simulink model "sistema_completo_OLD"  (R2023a)
settings: Solver=VariableStepAuto  StartTime=0.0  StopTime=2  MaxStep=1e-3  RelTol=1e-3
values from neighbouring files (symbols this model uses):
  Pp = 3    [angulo_de_desfasaje_electromagnetico.m]
  T_s_ref = 20    [Polos_ceros_Rs.m]
undefined symbols (not defined in the file or in its folder): alpha_Cu, b_eq, C_ts, J_eq, k_l, L_d, L_ls, L_q, lambda_m, omega_n_i, omega_n_pos, omega_n_v, r, R_s_ref, R_ts, tau, Vsl_max, zitta
libraries: SignalEditorBlockLib x9
settings Model: Creator=juanf  LastModifiedBy=Juan

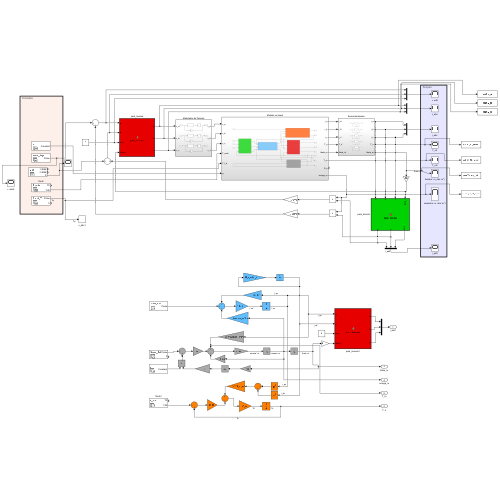
[thumbnail: Simulink's stored preview of the top-level diagram]
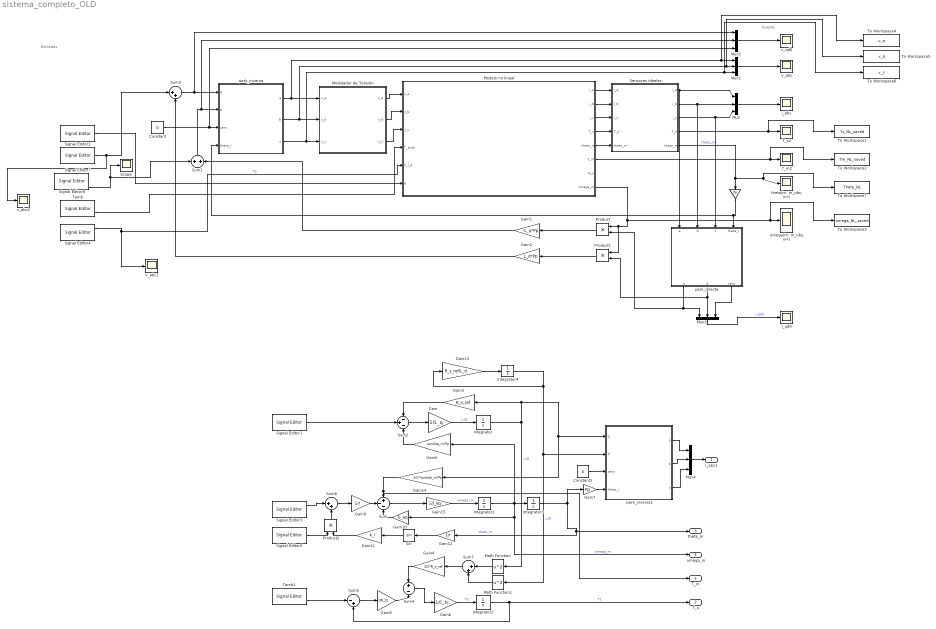
== system sistema_completo_OLD ==
  note: Scopes
  note: Entradas
  " " : Gain  Gain=Pp
  Constant : Constant  Value=0
  Constant1 : Constant  Value=0
  Gain : Gain  Gain=1/L_q
  Gain1 : Gain  Gain=-L_q*Pp
  Gain10 : Gain  Gain=b_eq
  Gain11 : Gain  Gain=k_l
  Gain12 : Gain  Gain=1/r
  Gain13 : Gain  Gain=R_s_ref/L_d
  Gain14 : Gain  Gain=3/2*lambda_m*Pp
  Gain15 : Gain  Gain=1/J_eq
  Gain2 : Gain  Gain=L_d*Pp
  Gain3 : Gain  Gain=R_s_ref
  Gain4 : Gain  Gain=3/2*R_s_ref
  Gain5 : Gain  Gain=lambda_m*Pp
  Gain6 : Gain  Gain=1/C_ts
  Gain7 : Gain  Gain=Pp
  Gain8 : Gain  Gain=1/R_ts
  Gain9 : Gain  Gain=1/r
  Integrator{,1,3..4} (4 alike) : Integrator
  Integrator2 : Integrator  InitialCondition=40
  Math Function : Math  Operator=square  SignedPower=on
  Math Function1 : Math  Operator=square  SignedPower=on
  Modelo no lineal : Subsystem
  Modulador de Tensión : Subsystem
  Mux{,1..4} (5 alike) : Mux  Inputs=3
  Product : Product
  Product1 : Product
  Product2 : Product
  Scope : Scope
  Sensores ideales : Subsystem
  Signal Editor1 : SignalEditorBlockLib/Signal Editor  FileName=D:\01. Facultad\AyME\Automatica-y-maquinas-electricas-final\Matlab - Simulink\señales\senal_Vqs.mat  ActiveScenario=senal_Vqs  ActiveSignal=Pulse  IsBus=off  OutputBusObjectStr=Bus: BusObject  SampleTime=0  Interpolate=off  ZeroCross=off  OutputAfterFinalValue=Setting to zero  Unit=inherit  PreserveSignalName=on  ApplySigPropsToAllScenarios=on
  Signal Editor2 : SignalEditorBlockLib/Signal Editor  FileName=D:\01. Facultad\AyME\Automatica-y-maquinas-electricas-final\Matlab - Simulink\señales\g.mat  ActiveScenario=g  ActiveSignal=Constant  IsBus=off  OutputBusObjectStr=Bus: BusObject  SampleTime=0  Interpolate=off  ZeroCross=off  OutputAfterFinalValue=Setting to zero  Unit=inherit  PreserveSignalName=on  ApplySigPropsToAllScenarios=on
  Signal Editor3 : SignalEditorBlockLib/Signal Editor  FileName=D:\01. Facultad\AyME\Automatica-y-maquinas-electricas-final\Matlab - Simulink\señales\senal_Tld.mat  ActiveScenario=Senal_Tld  ActiveSignal=Pulse  IsBus=off  OutputBusObjectStr=Bus: BusObject  SampleTime=0  Interpolate=off  ZeroCross=off  OutputAfterFinalValue=Setting to zero  Unit=inherit  PreserveSignalName=on  ApplySigPropsToAllScenarios=on
  Signal Editor4 : SignalEditorBlockLib/Signal Editor  FileName=D:\01. Facultad\AyME\Automatica-y-maquinas-electricas-final\Matlab - Simulink\señales\senal_Tld.mat  ActiveScenario=Senal_Tld  ActiveSignal=Pulse  IsBus=off  OutputBusObjectStr=Bus: BusObject  SampleTime=0  Interpolate=off  ZeroCross=off  OutputAfterFinalValue=Setting to zero  Unit=inherit  PreserveSignalName=on  ApplySigPropsToAllScenarios=on
  Signal Editor6 : SignalEditorBlockLib/Signal Editor  FileName=D:\01. Facultad\AyME\Automatica-y-maquinas-electricas-final\Matlab - Simulink\señales\g.mat  ActiveScenario=g  ActiveSignal=Constant  IsBus=off  OutputBusObjectStr=Bus: BusObject  SampleTime=0  Interpolate=off  ZeroCross=off  OutputAfterFinalValue=Setting to zero  Unit=inherit  PreserveSignalName=on  ApplySigPropsToAllScenarios=on
  Signal Editor7 : SignalEditorBlockLib/Signal Editor  FileName=D:\01. Facultad\AyME\Automatica-y-maquinas-electricas-final\Matlab - Simulink\señales\senal_Vqs.mat  ActiveScenario=senal_Vqs  ActiveSignal=Pulse  IsBus=off  OutputBusObjectStr=Bus: BusObject  SampleTime=0  Interpolate=off  ZeroCross=off  OutputAfterFinalValue=Setting to zero  Unit=inherit  PreserveSignalName=on  ApplySigPropsToAllScenarios=on
  Signal Editor8 : SignalEditorBlockLib/Signal Editor  FileName=D:\01. Facultad\AyME\Automatica-y-maquinas-electricas-final\Matlab - Simulink\señales\V_d.mat  ActiveScenario=V_d  ActiveSignal=1.9596  IsBus=off  OutputBusObjectStr=Bus: BusObject  SampleTime=0  Interpolate=off  ZeroCross=off  OutputAfterFinalValue=Setting to zero  Unit=inherit  PreserveSignalName=on  ApplySigPropsToAllScenarios=on
  Sin : Trigonometry
  Sum : Sum  Inputs=+--
  Sum1 : Sum  Inputs=+|+
  Sum2 : Sum  Inputs=-+-
  Sum3 : Sum  Inputs=|++
  Sum4 : Sum  Inputs=+|-
  Sum5 : Sum  Inputs=|-+
  Sum6 : Sum  Inputs=|++
  Sum7 : Sum  Inputs=|++
  T_m2 : Scope
  T_s2 : Scope
  Tamb : SignalEditorBlockLib/Signal Editor  FileName=D:\01. Facultad\AyME\Automatica-y-maquinas-electricas-final\Matlab - Simulink\señales\senal_Tamb.mat  ActiveScenario=T_amb  ActiveSignal=T0  IsBus=off  OutputBusObjectStr=Bus: BusObject  SampleTime=0  Interpolate=off  ZeroCross=off  OutputAfterFinalValue=Setting to zero  Unit=inherit  PreserveSignalName=on  ApplySigPropsToAllScenarios=on
  Tamb1 : SignalEditorBlockLib/Signal Editor  FileName=D:\01. Facultad\AyME\Automatica-y-maquinas-electricas-final\Matlab - Simulink\señales\senal_Tamb.mat  ActiveScenario=T_amb  ActiveSignal=T0  IsBus=off  OutputBusObjectStr=Bus: BusObject  SampleTime=0  Interpolate=off  ZeroCross=off  OutputAfterFinalValue=Setting to zero  Unit=inherit  PreserveSignalName=on  ApplySigPropsToAllScenarios=on
  To Workspace1 : ToWorkspace  VariableName=Ts_NL_saved  SaveFormat=Timeseries  SampleTime=-1
  To Workspace2 : ToWorkspace  VariableName=Tm_NL_saved  SaveFormat=Timeseries  SampleTime=-1
  To Workspace3 : ToWorkspace  VariableName=omega_NL_saved  SaveFormat=Timeseries  SampleTime=-1
  To Workspace4 : ToWorkspace  VariableName=v_a  SaveFormat=Timeseries  SampleTime=-1
  To Workspace5 : ToWorkspace  VariableName=v_b  SaveFormat=Timeseries  SampleTime=-1
  To Workspace6 : ToWorkspace  VariableName=v_c  SaveFormat=Timeseries  SampleTime=-1
  To Workspace7 : ToWorkspace  VariableName=Theta_NL  SaveFormat=Timeseries  SampleTime=-1
  i_abc : Scope
  i_qd0 : Scope
  omega(m; m_obs; m*) : Scope
  park_directa : MATLAB Function  TreatAsAtomicUnit=on
  park_inversa : MATLAB Function  TreatAsAtomicUnit=on
  park_inversa1 : MATLAB Function  TreatAsAtomicUnit=on
  theta(m; m_obs; m*) : Scope
  v_abc : Scope
  v_abc1 : Scope
  v_abc2 : Scope
  v_qd0 : Scope
  i_abc1 : Outport
  T_s : Outport  Port=2
  theta_m : Outport  Port=3
  omega_m : Outport  Port=4
  T_m : Outport  Port=5
  wires:
  park_inversa/1(a) -> To Workspace4/1, Mux1/1, Modulador de Tensión/1(v_a)
  park_inversa/2(b) -> To Workspace5/1, Mux1/2, Modulador de Tensión/2(v_b)
  park_inversa/3(c) -> To Workspace6/1, Mux1/3, Modulador de Tensión/3(v_c)
  Modulador de Tensión/1(v_a') -> Modelo no lineal/1(v_a)
  Modulador de Tensión/2(v_b') -> Modelo no lineal/2(v_b)
  Modulador de Tensión/3(v_c') -> Modelo no lineal/3(v_c)
  Modelo no lineal/1(i_a) -> Sensores ideales/1(i_a')
  Modelo no lineal/2(i_b) -> Sensores ideales/2(i_b')
  Modelo no lineal/3(i_c) -> Sensores ideales/3(i_c')
  Modelo no lineal/4(T_s) -> Sensores ideales/4(T_s')
  Modelo no lineal/5(theta_m) -> Sensores ideales/5(theta_m')
  Modelo no lineal/6(T_m) -> To Workspace2/1, T_m2/1
  Sensores ideales/1(i_a) -> Mux/1, park_directa/1(a)
  Sensores ideales/2(i_b) -> Mux/2, park_directa/2(b)
  Sensores ideales/3(i_c) -> Mux/3, park_directa/3(c)
  Modelo no lineal/8(omega_m) -> Product1/1, Product/1, To Workspace3/1, omega(m; m_obs; m*)/1
  Sum3/1 -> Mux2/1, park_inversa/1(q)
  Sensores ideales/4(T_s) -> To Workspace1/1, T_s2/1
  park_directa/1(q) -> Product/2, Mux3/1
  park_directa/2(d) -> Mux3/2, Product1/2
  park_directa/3(zero) -> Mux3/3
  " "/1 -> park_inversa/4(theta_r), park_directa/4(theta_r)
  Product/1 -> Gain1/1
  Mux/1 -> i_abc/1
  Mux2/1 -> v_qd0/1
  Mux3/1 -> i_qd0/1  "i_qd0"
  Sum1/1 -> Mux2/2, park_inversa/2(d)
  Product1/1 -> Gain2/1
  Gain2/1 -> Sum3/2
  Gain1/1 -> Sum1/2
  Signal Editor7/1 -> v_abc2/1, Sum3/1
  Constant/1 -> Mux2/3, park_inversa/3(zero)
  Signal Editor8/3 -> Scope/1, Sum1/1
  Gain3/1 -> Sum2/1
  Integrator/1 -> park_inversa1/1(q), Gain14/1, Gain3/1, Math Function/1  "i_qs"
  park_inversa1/1(a) -> Mux4/1
  park_inversa1/3(c) -> Mux4/3
  Sum6/1 -> Gain9/1
  Sum/1 -> Gain15/1
  Integrator4/1 -> Gain13/1, Math Function1/1, park_inversa1/2(d)  "i_ds"
  Sin/1 -> Gain11/1
  park_inversa1/2(b) -> Mux4/2
  Sum7/1 -> Gain4/1
  Math Function1/1 -> Sum7/2
  Gain6/1 -> Integrator2/1  "Ts'"
  Integrator2/1 -> Sum5/2, T_s/1  "Ts"
  Gain13/1 -> Integrator4/1
  Mux4/1 -> i_abc1/1
  Signal Editor6/1 -> Product2/1
  Gain15/1 -> Integrator1/1  "omega'_m"
  Tamb1/2 -> Sum5/1
  Math Function/1 -> Sum7/1
  Gain14/1 -> Sum/1, T_m/1
  Gain7/1 -> park_inversa1/4(theta_r)
  Sum2/1 -> Gain/1
  Gain/1 -> Integrator/1  "i_qs'"
  Constant1/1 -> park_inversa1/3(zero)
  Gain4/1 -> Sum4/1
  Gain11/1 -> Product2/2
  Signal Editor3/1 -> Sum6/1
  Sum4/1 -> Gain6/1
  Signal Editor1/1 -> Sum2/2
  Product2/1 -> Sum6/2
  Sum5/1 -> Gain8/1
  Integrator3/1 -> Gain12/1, theta_m/1, Gain7/1  "theta_m"
  Gain9/1 -> Sum/2
  Gain10/1 -> Sum/3
  Gain12/1 -> Sin/1
  Gain5/1 -> Sum2/3
  Gain8/1 -> Sum4/2
  Integrator1/1 -> omega_m/1, Gain10/1, Integrator3/1, Gain5/1  "omega_m"
  Tamb/2 -> Modelo no lineal/4(T_amb)
  Signal Editor4/1 -> Modelo no lineal/5(T_l_d), v_abc1/1  "Tp"
  Signal Editor2/1 -> Modelo no lineal/6(g)
  Mux1/1 -> v_abc/1
  Sensores ideales/5(theta_m) -> " "/1, To Workspace7/1, theta(m; m_obs; m*)/1  "theta_m"

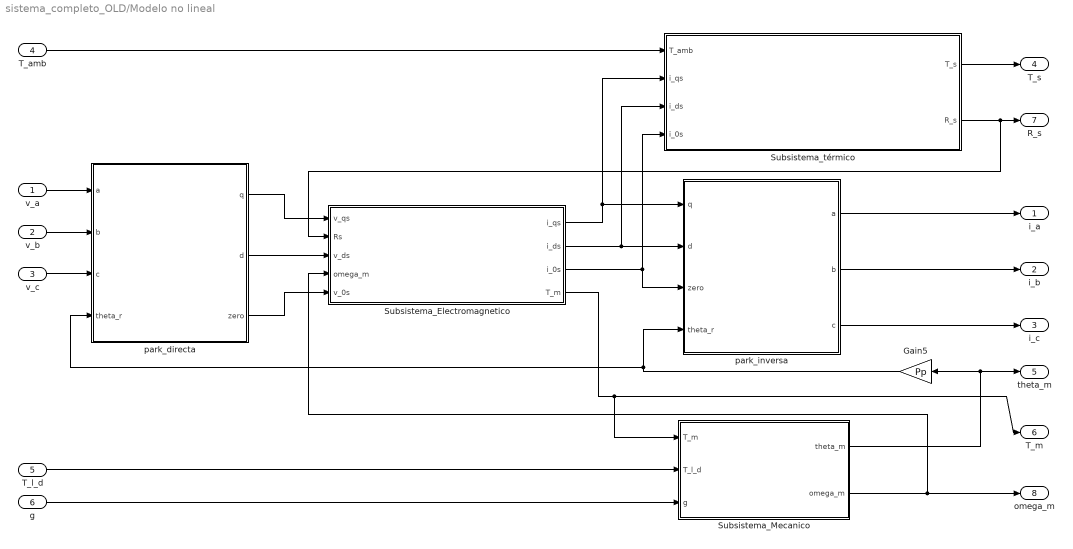
== system sistema_completo_OLD/Modelo no lineal ==
  v_a : Inport
  v_b : Inport  Port=2
  v_c : Inport  Port=3
  T_amb : Inport  Port=4
  T_l_d : Inport  Port=5
  g : Inport  Port=6
  Gain5 : Gain  Gain=Pp
  Subsistema_Electromagnetico : Subsystem
  Subsistema_Mecanico : Subsystem
  Subsistema_térmico : Subsystem
  park_directa : MATLAB Function  TreatAsAtomicUnit=on
  park_inversa : MATLAB Function  TreatAsAtomicUnit=on
  i_a : Outport
  i_b : Outport  Port=2
  i_c : Outport  Port=3
  T_s : Outport  Port=4
  theta_m : Outport  Port=5
  T_m : Outport  Port=6
  R_s : Outport  Port=7
  omega_m : Outport  Port=8
  wires:
  v_b/1 -> park_directa/2(b)
  Subsistema_Mecanico/1(theta_m) -> theta_m/1, Gain5/1
  T_l_d/1 -> Subsistema_Mecanico/2(T_l_d)
  park_directa/2(d) -> Subsistema_Electromagnetico/3(v_ds)
  Subsistema_Electromagnetico/4(T_m) -> Subsistema_Mecanico/1(T_m), T_m/1
  T_amb/1 -> Subsistema_térmico/1(T_amb)
  Subsistema_térmico/1(T_s) -> T_s/1
  Gain5/1 -> park_directa/4(theta_r), park_inversa/4(theta_r)
  v_a/1 -> park_directa/1(a)
  Subsistema_Mecanico/2(omega_m) -> omega_m/1, Subsistema_Electromagnetico/4(omega_m)
  park_directa/1(q) -> Subsistema_Electromagnetico/1(v_qs)
  Subsistema_térmico/2(R_s) -> Subsistema_Electromagnetico/2(Rs), R_s/1
  v_c/1 -> park_directa/3(c)
  park_inversa/2(b) -> i_b/1
  Subsistema_Electromagnetico/2(i_ds) -> park_inversa/2(d), Subsistema_térmico/3(i_ds)
  park_inversa/1(a) -> i_a/1
  Subsistema_Electromagnetico/1(i_qs) -> park_inversa/1(q), Subsistema_térmico/2(i_qs)
  park_inversa/3(c) -> i_c/1
  Subsistema_Electromagnetico/3(i_0s) -> park_inversa/3(zero), Subsistema_térmico/4(i_0s)
  park_directa/3(zero) -> Subsistema_Electromagnetico/5(v_0s)
  g/1 -> Subsistema_Mecanico/3(g)

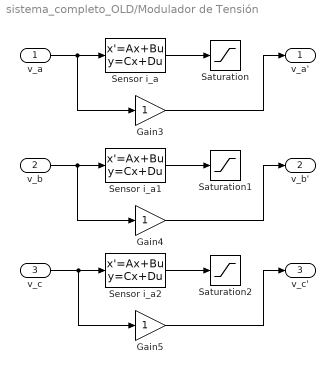
== system sistema_completo_OLD/Modulador de Tensión ==
  v_a : Inport
  v_b : Inport  Port=2
  v_c : Inport  Port=3
  Gain3 : Gain
  Gain4 : Gain
  Gain5 : Gain
  Saturation : Saturate  UpperLimit=Vsl_max  LowerLimit=-Vsl_max
  Saturation1 : Saturate  UpperLimit=Vsl_max  LowerLimit=-Vsl_max
  Saturation2 : Saturate  UpperLimit=Vsl_max  LowerLimit=-Vsl_max
  Sensor i_a : StateSpace  A=[0 1 ; -omega_n_v^2 -2*zitta*omega_n_v]  B=[0; omega_n_v^2]  C=[1 0]  D=[0]  InitialCondition=0  AllowTunableDMatrix=on
  Sensor i_a1 : StateSpace  A=[0 1 ; -omega_n_v^2 -2*zitta*omega_n_v]  B=[0; omega_n_v^2]  C=[1 0]  D=[0]  InitialCondition=0  AllowTunableDMatrix=on
  Sensor i_a2 : StateSpace  A=[0 1 ; -omega_n_v^2 -2*zitta*omega_n_v]  B=[0; omega_n_v^2]  C=[1 0]  D=[0]  InitialCondition=0  AllowTunableDMatrix=on
  v_a' : Outport
  v_b' : Outport  Port=2
  v_c' : Outport  Port=3
  wires:
  v_b/1 -> Sensor i_a1/1, Gain4/1
  v_a/1 -> Gain3/1, Sensor i_a/1
  Sensor i_a1/1 -> Saturation1/1
  Sensor i_a2/1 -> Saturation2/1
  v_c/1 -> Sensor i_a2/1, Gain5/1
  Sensor i_a/1 -> Saturation/1
  Gain5/1 -> v_c'/1
  Gain4/1 -> v_b'/1
  Gain3/1 -> v_a'/1

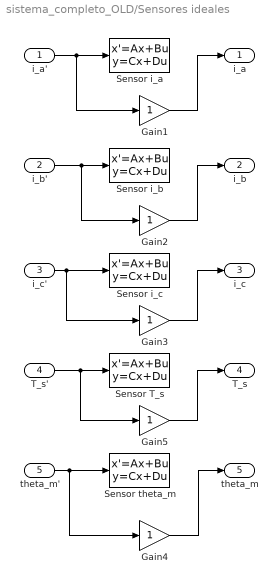
== system sistema_completo_OLD/Sensores ideales ==
  i_a' : Inport
  i_b' : Inport  Port=2
  i_c' : Inport  Port=3
  T_s' : Inport  Port=4
  theta_m' : Inport  Port=5
  Gain{1..5} (5 alike) : Gain
  Sensor T_s : StateSpace  A=[-1/tau]  B=[1/tau]  C=[1]  D=[0]  InitialCondition=40  AllowTunableDMatrix=on
  Sensor i_a : StateSpace  A=[0 1 ; -omega_n_i^2 -2*zitta*omega_n_i]  B=[0; omega_n_i^2]  C=[1 0]  D=[0]  InitialCondition=0  AllowTunableDMatrix=on
  Sensor i_b : StateSpace  A=[0 1 ; -omega_n_i^2 -2*zitta*omega_n_i]  B=[0; omega_n_i^2]  C=[1 0]  D=[0]  InitialCondition=0  AllowTunableDMatrix=on
  Sensor i_c : StateSpace  A=[0 1 ; -omega_n_i^2 -2*zitta*omega_n_i]  B=[0; omega_n_i^2]  C=[1 0]  D=[0]  InitialCondition=0  AllowTunableDMatrix=on
  Sensor theta_m : StateSpace  A=[0 1 ; -omega_n_pos^2 -2*zitta*omega_n_pos]  B=[0; omega_n_pos^2]  C=[1 0]  D=[0]  InitialCondition=0  AllowTunableDMatrix=on
  i_a : Outport
  i_b : Outport  Port=2
  i_c : Outport  Port=3
  T_s : Outport  Port=4
  theta_m : Outport  Port=5
  wires:
  i_a'/1 -> Gain1/1, Sensor i_a/1
  i_b'/1 -> Gain2/1, Sensor i_b/1
  i_c'/1 -> Gain3/1, Sensor i_c/1
  T_s'/1 -> Gain5/1, Sensor T_s/1
  theta_m'/1 -> Gain4/1, Sensor theta_m/1
  Gain1/1 -> i_a/1
  Gain2/1 -> i_b/1
  Gain3/1 -> i_c/1
  Gain5/1 -> T_s/1
  Gain4/1 -> theta_m/1

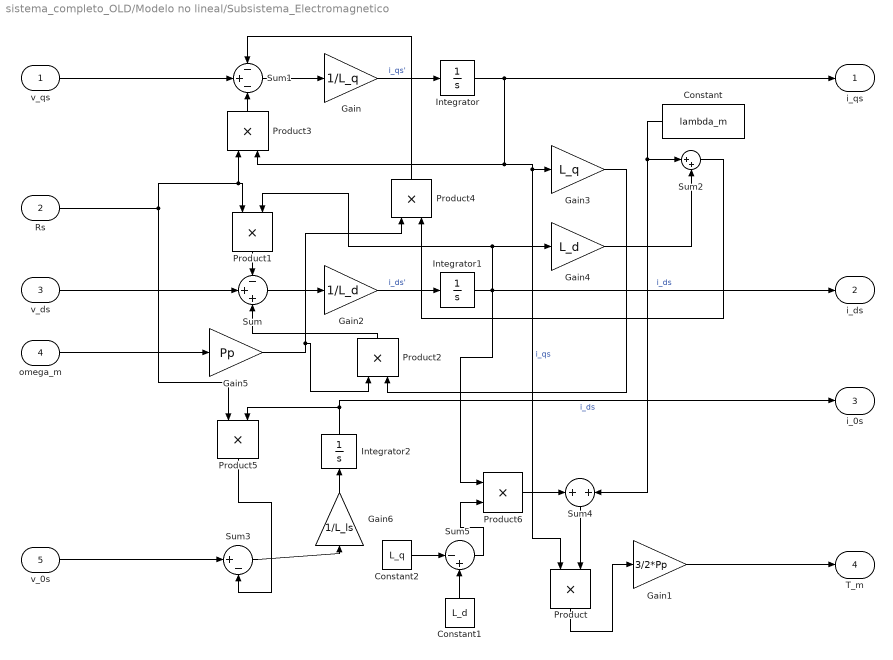
== system sistema_completo_OLD/Modelo no lineal/Subsistema_Electromagnetico ==
  v_qs : Inport
  Rs : Inport  Port=2
  v_ds : Inport  Port=3
  omega_m : Inport  Port=4
  v_0s : Inport  Port=5
  Constant : Constant  Value=lambda_m
  Constant1 : Constant  Value=L_d
  Constant2 : Constant  Value=L_q
  Gain : Gain  Gain=1/L_q
  Gain1 : Gain  Gain=3/2*Pp
  Gain2 : Gain  Gain=1/L_d
  Gain3 : Gain  Gain=L_q
  Gain4 : Gain  Gain=L_d
  Gain5 : Gain  Gain=Pp
  Gain6 : Gain  Gain=1/L_ls
  Integrator : Integrator
  Integrator1 : Integrator
  Integrator2 : Integrator
  Product{,1..6} (7 alike) : Product
  Sum : Sum  Inputs=-++
  Sum1 : Sum  Inputs=-+-
  Sum2 : Sum  Inputs=|++
  Sum3 : Sum  Inputs=|+-
  Sum4 : Sum
  Sum5 : Sum  Inputs=|-+
  i_qs : Outport
  i_ds : Outport  Port=2
  i_0s : Outport  Port=3
  T_m : Outport  Port=4
  wires:
  Gain1/1 -> T_m/1
  Product/1 -> Gain1/1
  v_qs/1 -> Sum1/2
  Sum1/1 -> Gain/1
  Gain/1 -> Integrator/1  "i_qs'"
  Integrator/1 -> Product/1, Gain3/1, Product3/2, i_qs/1  "i_qs"
  Product3/1 -> Sum1/3
  Rs/1 -> Product3/1, Product1/1, Product5/1
  Product4/1 -> Sum1/1
  Product1/1 -> Sum/1
  v_ds/1 -> Sum/2
  Sum/1 -> Gain2/1
  Gain2/1 -> Integrator1/1  "i_ds'"
  Integrator1/1 -> i_ds/1, Product6/1, Gain4/1, Product1/2  "i_ds"
  Constant/1 -> Sum4/2, Sum2/1
  Sum2/1 -> Product4/2
  omega_m/1 -> Gain5/1
  Gain5/1 -> Product2/1, Product4/1
  Product2/1 -> Sum/3
  Gain4/1 -> Sum2/2
  Gain3/1 -> Product2/2
  v_0s/1 -> Sum3/1
  Product5/1 -> Sum3/2
  Sum3/1 -> Gain6/1
  Gain6/1 -> Integrator2/1
  Integrator2/1 -> Product5/2, i_0s/1  "i_ds"
  Constant1/1 -> Sum5/2
  Constant2/1 -> Sum5/1
  Product6/1 -> Sum4/1
  Sum5/1 -> Product6/2
  Sum4/1 -> Product/2

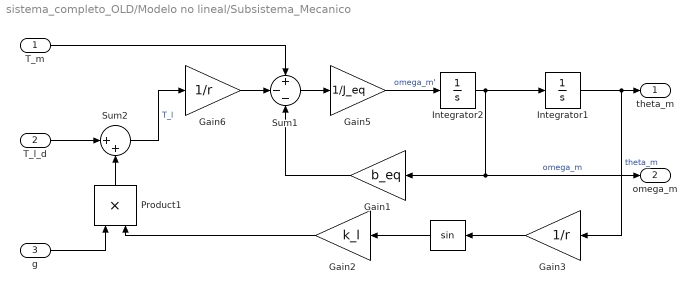
== system sistema_completo_OLD/Modelo no lineal/Subsistema_Mecanico ==
  T_m : Inport
  T_l_d : Inport  Port=2
  g : Inport  Port=3
  " " : Trigonometry
  Gain1 : Gain  Gain=b_eq
  Gain2 : Gain  Gain=k_l
  Gain3 : Gain  Gain=1/r
  Gain5 : Gain  Gain=1/J_eq
  Gain6 : Gain  Gain=1/r
  Integrator1 : Integrator
  Integrator2 : Integrator
  Product1 : Product
  Sum1 : Sum  Inputs=+--
  Sum2 : Sum  Inputs=|++
  theta_m : Outport
  omega_m : Outport  Port=2
  wires:
  T_l_d/1 -> Sum2/1
  Integrator1/1 -> Gain3/1, theta_m/1  "theta_m"
  Gain3/1 -> " "/1
  " "/1 -> Gain2/1
  Gain1/1 -> Sum1/3
  Sum1/1 -> Gain5/1
  Sum2/1 -> Gain6/1  "T_l"
  Gain6/1 -> Sum1/2
  Integrator2/1 -> Integrator1/1, Gain1/1, omega_m/1  "omega_m"
  Gain5/1 -> Integrator2/1  "omega_m'"
  Gain2/1 -> Product1/2
  T_m/1 -> Sum1/1
  g/1 -> Product1/1
  Product1/1 -> Sum2/2

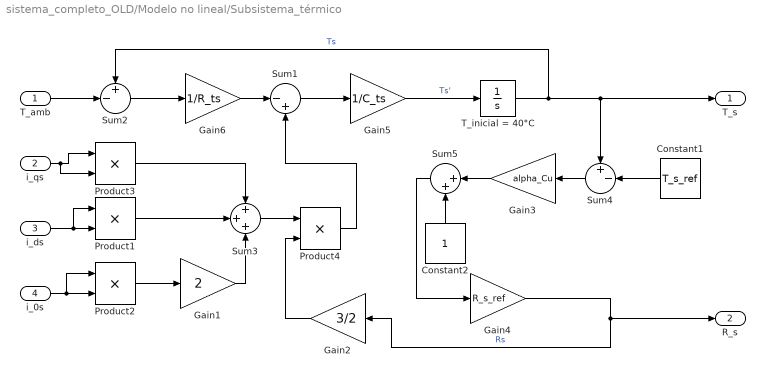
== system sistema_completo_OLD/Modelo no lineal/Subsistema_térmico ==
  T_amb : Inport
  i_qs : Inport  Port=2
  i_ds : Inport  Port=3
  i_0s : Inport  Port=4
  Constant1 : Constant  Value=T_s_ref
  Constant2 : Constant
  Gain1 : Gain  Gain=2
  Gain2 : Gain  Gain=3/2
  Gain3 : Gain  Gain=alpha_Cu
  Gain4 : Gain  Gain=R_s_ref
  Gain5 : Gain  Gain=1/C_ts
  Gain6 : Gain  Gain=1/R_ts
  Product{1..4} (4 alike) : Product
  Sum1 : Sum  Inputs=|-+
  Sum2 : Sum  Inputs=+-|
  Sum3 : Sum  Inputs=+++
  Sum4 : Sum  Inputs=+-|
  Sum5 : Sum  Inputs=|++
  T_inicial = 40°C : Integrator  InitialCondition=40
  T_s : Outport
  R_s : Outport  Port=2
  wires:
  Gain5/1 -> T_inicial = 40°C/1  "Ts'"
  Sum1/1 -> Gain5/1
  Sum2/1 -> Gain6/1
  T_amb/1 -> Sum2/2
  T_inicial = 40°C/1 -> Sum4/1, T_s/1, Sum2/1  "Ts"
  i_qs/1 -> Product3/2, Product3/1
  i_0s/1 -> Product2/1, Product2/2
  Product2/1 -> Gain1/1
  Gain1/1 -> Sum3/3
  Product1/1 -> Sum3/2
  Product3/1 -> Sum3/1
  Sum3/1 -> Product4/1
  Gain2/1 -> Product4/2
  Gain6/1 -> Sum1/1
  Product4/1 -> Sum1/2
  Constant1/1 -> Sum4/2
  Sum4/1 -> Gain3/1
  Constant2/1 -> Sum5/2
  Sum5/1 -> Gain4/1
  Gain4/1 -> Gain2/1, R_s/1  "Rs"
  Gain3/1 -> Sum5/1
  i_ds/1 -> Product1/2, Product1/1

== matlab function sistema_completo_OLD/park_inversa ==
  data: q input; a output; d input; zero input; theta_r input; b output; c output
function [a, b, c] = park_inversa(q, d, zero, theta_r)
% qd0 → abc (transformacion inversa)
% Entradas: q, d, zero (coordenadas qd0), theta_r (ángulo eléctrico)
% Salidas: a, b, c (señales de fase)
    
    T_inv = [cos(theta_r),               sin(theta_r),              1;
             cos(theta_r - 2*pi/3),      sin(theta_r - 2*pi/3),     1;
             cos(theta_r + 2*pi/3),      sin(theta_r + 2*pi/3),     1];
    
    abc = T_inv * [q; d; zero];

    a = abc(1);
    b = abc(2);
    c = abc(3);
end

== matlab function sistema_completo_OLD/park_directa ==
  data: a input; q output; b input; c input; theta_r input; d output; zero output
function [q, d, zero] = park_directa(a, b, c, theta_r)
% Transformacion abc → qd0
% a, b y c son señales de fase y theta_r es el angulo ELECTRICO (no mecanico) del rotor)
% Salidas: q, d, zero, que son las coordenadas virtuales qd0
    
    T = (2/3) * [cos(theta_r),           cos(theta_r - 2*pi/3),      cos(theta_r + 2*pi/3);
                 sin(theta_r),           sin(theta_r - 2*pi/3),      sin(theta_r + 2*pi/3);
                 1/2,                    1/2,                         1/2];
    
    qd0 = T * [a; b; c];
    
% asignar salidas
    q = qd0(1);
    d = qd0(2);
    zero = qd0(3);
end

== matlab function sistema_completo_OLD/Modelo no lineal/park_directa ==
  data: a input; q output; b input; c input; theta_r input; d output; zero output
function [q, d, zero] = park_directa(a, b, c, theta_r)
% Transformacion abc → qd0
% a, b y c son señales de fase y theta_r es el angulo ELECTRICO (no mecanico) del rotor)
% Salidas: q, d, zero, que son las coordenadas virtuales qd0
    
    T = (2/3) * [cos(theta_r),           cos(theta_r - 2*pi/3),      cos(theta_r + 2*pi/3);
                 sin(theta_r),           sin(theta_r - 2*pi/3),      sin(theta_r + 2*pi/3);
                 1/2,                    1/2,                         1/2];
    
    qd0 = T * [a; b; c];
    
% asignar salidas
    q = qd0(1);
    d = qd0(2);
    zero = qd0(3);
end

== matlab function sistema_completo_OLD/Modelo no lineal/park_inversa ==
  data: q input; a output; d input; zero input; theta_r input; b output; c output
function [a, b, c] = park_inversa(q, d, zero, theta_r)
% qd0 → abc (transformacion inversa)
% Entradas: q, d, zero (coordenadas qd0), theta_r (ángulo eléctrico)
% Salidas: a, b, c (señales de fase)
    
    T_inv = [cos(theta_r),               sin(theta_r),              1;
             cos(theta_r - 2*pi/3),      sin(theta_r - 2*pi/3),     1;
             cos(theta_r + 2*pi/3),      sin(theta_r + 2*pi/3),     1];
    
    abc = T_inv * [q; d; zero];

    a = abc(1);
    b = abc(2);
    c = abc(3);
end

== matlab function sistema_completo_OLD/park_inversa1 ==
  data: q input; a output; d input; zero input; theta_r input; b output; c output
function [a, b, c] = park_inversa(q, d, zero, theta_r)
% qd0 → abc (transformacion inversa)
% Entradas: q, d, zero (coordenadas qd0), theta_r (ángulo eléctrico)
% Salidas: a, b, c (señales de fase)
    
    T_inv = [cos(theta_r),               sin(theta_r),              1;
             cos(theta_r - 2*pi/3),      sin(theta_r - 2*pi/3),     1;
             cos(theta_r + 2*pi/3),      sin(theta_r + 2*pi/3),     1];
    
    abc = T_inv * [q; d; zero];

    a = abc(1);
    b = abc(2);
    c = abc(3);
end
